simulink model "rocky_motor_disturb_pid"  (R2020a)
settings: Solver=VariableStepAuto  StartTime=0.0  StopTime=2  RelTol=1e-3
model workspace (MAT data in the model file):
  m = 1000
undefined symbols (not defined in the file): Ci, g, Jicp, Jp, Ki, kmotor, Kp, l, tau
settings Model: Creator=clee1  LastModifiedBy=lila

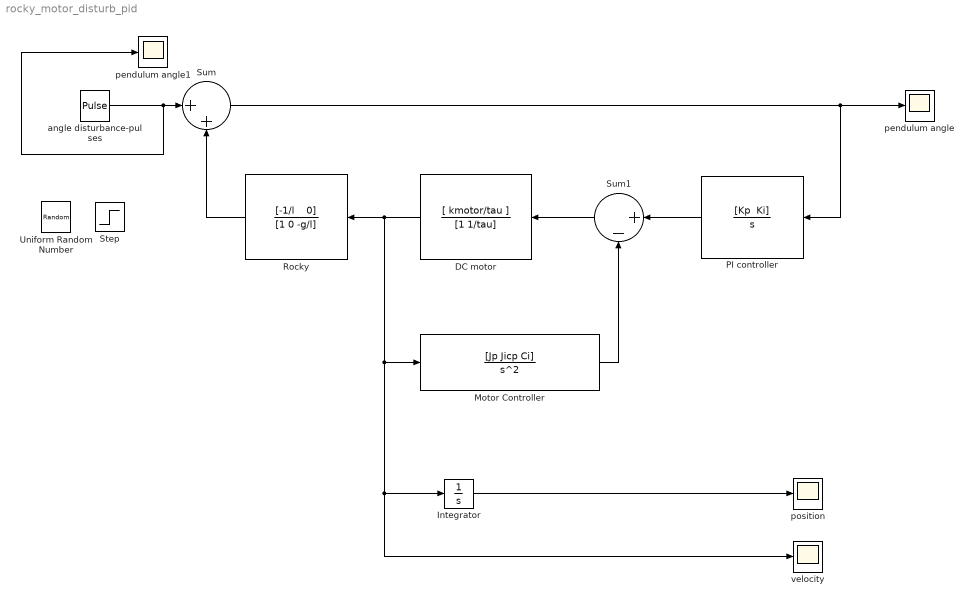
== system rocky_motor_disturb_pid ==
  DC motor : TransferFcn  Numerator=[ kmotor/tau ]  Denominator=[1 1/tau]
  Integrator : Integrator
  Motor Controller : TransferFcn  Numerator=[Jp Jicp Ci]  Denominator=[1 0 0]
  PI controller : TransferFcn  Numerator="[Kp  Ki]"  Denominator=[1 0 ]
  Rocky : TransferFcn  Numerator="[-1/l    0]"  Denominator=[1 0 -g/l]
  Step : Step  After=.1  SampleTime=0
  Sum : Sum  Inputs=|++
  Sum1 : Sum  Inputs=|+-
  Uniform Random Number : UniformRandomNumber  SampleTime=20
  angle disturbance-pulses : DiscretePulseGenerator  PulseType=Time based  Amplitude=.1  Period=10  PulseWidth=.1  PhaseDelay=.5
  pendulum angle : Scope
  pendulum angle1 : Scope
  position : Scope
  "velocity " : Scope
  wires:
  Rocky/1 -> Sum/2
  Sum/1 -> PI controller/1, pendulum angle/1
  angle disturbance-pulses/1 -> pendulum angle1/1, Sum/1
  DC motor/1 -> "velocity "/1, Integrator/1, Motor Controller/1, Rocky/1
  Integrator/1 -> position/1
  PI controller/1 -> Sum1/1
  Sum1/1 -> DC motor/1
  Motor Controller/1 -> Sum1/2
